simulink model "sampleModel1647"  (R2023a)
settings: Solver=VariableStepAuto  StartTime=0.0  StopTime=10.0  RelTol=1e-3
libraries: hdlsllib x7, simulink x4
settings Model: Creator=user1  LastModifiedBy=user1

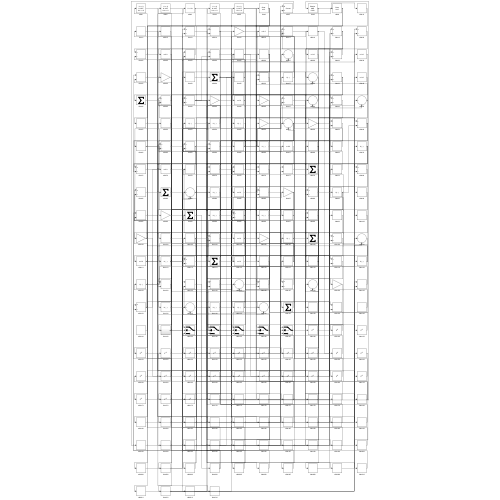
[thumbnail: Simulink's stored preview of the top-level diagram]
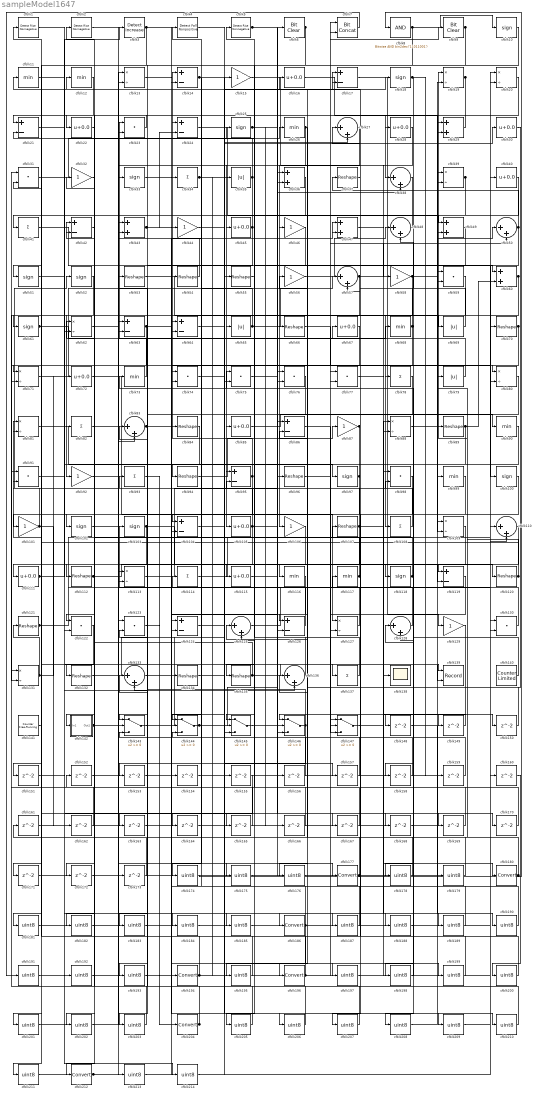
== system sampleModel1647 ==
  cfblk1 : hdlsllib/Logic and Bit Operations/Detect Rise Nonnegative  vinit=0  OutDataTypeStr=boolean
  cfblk{10,18,25,33,51..52,61,97,100,102..103,118} (12 alike) : Signum
  cfblk{15,32,44,46,56,58,87,92,101,106,129} (11 alike) : Gain
  cfblk{14,17,21,24,42,63..64,86,95,104,119,124,126} (13 alike) : Sum  Inputs=+-
  cfblk{16,22,28,30,40,45,67,72,85,105,111,115} (12 alike) : Bias  Bias=0.0  SaturateOnIntegerOverflow=off
  cfblk{37,53..55,66,70,84,89,94,96,107,112,120..121,132,134..135} (17 alike) : Reshape
  cfblk{34,41,78,82,93,108,114,137} (8 alike) : Sum  Inputs=+
  cfblk{13,19..20,39,62,71,80..81,88,109,113,127,131} (13 alike) : Product  Inputs=*/  RndMeth=Zero  SaturateOnIntegerOverflow=on
  cfblk{11..12,26,68,73,90,99,116..117} (9 alike) : MinMax
  cfblk{27,38,48,50,57,83,110,125,128,133,136} (11 alike) : Sum  Inputs=|++
  cfblk{23,31,59,74..77,91,98,122..123,130} (12 alike) : DotProduct  OutDataTypeStr=Inherit: Inherit via internal rule
  cfblk138 : Scope
  cfblk139 : Record  FileSettingsInternal="{\"entries\":[{\"content\":{\"excelSettings\":{\"content\":{},\"type\":\"Streamout.ExcelSettings\"}},\"type\":\"Streamout.FileSettingStorage\",\"uuid\":\"\"}],\"packageUris\":[\"http:\\/\\/schema.mathworks.com\\/mf0\\/streamout_blocks\\/R2020a\"],\"version\":\"1.0\"}"  Layout=[1 1]  SignalsInternal="{\"entries\":[{\"content\":{\"signals\":[{\"content\":{\"blockPath\":[],\"dimensions\":[1],\"domain\":\"\",\"lineColor\":\"#a2142f\",\"plots\":[1],\"port\":1,\"signalID\":2509,\"signalName\":\"XY Graph:1\"},\"type\":\"RecordBlkView.Signal\",\"uuid\":\"\"},{\"content\":{\"blockPath\":[],\"dimensions\":[1],\"domain\":\"\",\"lineColor\":\"#139fff\",\"plots\":[1],\"port\":2,\"signalID\":2512,\"signalName\":\"XY Graph:2\"},\"type\":\"RecordBlkView.Signal\",\"uuid\":\"\"}]},\"type\":\"RecordBlkView.InputSignals\",\"uuid\":\"\"}],\"packageUris\":[\"http:\\/\\/schema.mathworks.com\\/mf0\\/streamout_blocks\\/R2020a\"],\"version\":\"1.0\"}"  VisualizationBindings="{\"xyplotplugin\":{\"info\":[{\"series\":[{\"bindingParametersList\":[{\"parameter\":\"X-Axis\",\"signalID\":2509,\"signalName\":\"XY Graph:1\"},{\"parameter\":\"Y-Axis\",\"signalID\":2512,\"signalName\":\"XY Graph:2\"}],\"seriesID\":52686}],\"subplotID\":1}]}}"  CompatibilityTag=XY  st=-1
  cfblk140 : hdlsllib/Sources/Counter Limited  uplimit=7  tsamp=-1
  cfblk141 : hdlsllib/Sources/Counter Free-Running  NumBits=16  tsamp=-1
  cfblk142 : Subsystem
      settings: LibrarySourceBlock=|
      | hdlsllib/Ports &
      | Subsystems/Subsystem
  cfblk{143..147} (5 alike) : Switch  SaturateOnIntegerOverflow=off  InputSameDT=off
  cfblk{148..173} (26 alike) : Delay  SampleTime=1
  cfblk{174..176,178..179,181..185,187..193,195,197..203,205..211,213..214} (34 alike) : DataTypeConversion  OutDataTypeStr=uint8  SaturateOnIntegerOverflow=off  RndMeth=Floor
  cfblk{177,180,186,194,196,204,212} (7 alike) : DataTypeConversion  SaturateOnIntegerOverflow=off  RndMeth=Floor
  cfblk2 : hdlsllib/Logic and Bit Operations/Detect Rise Nonnegative  vinit=0  OutDataTypeStr=boolean
  cfblk{29,36,43,47,49,60} (6 alike) : Sum
  cfblk3 : simulink/Logic and Bit Operations/Detect Increase  vinit=0.0  OutDataTypeStr=boolean
      settings: LibrarySourceBlock=|
      | hdlsllib/Logic and Bit
      | Operations/Detect
      | Increase
  cfblk{35,65,69,79} (4 alike) : Abs  SaturateOnIntegerOverflow=off
  cfblk4 : hdlsllib/Logic and Bit Operations/Detect Fall Nonpositive  vinit=0  OutDataTypeStr=boolean
  cfblk5 : hdlsllib/Logic and Bit Operations/Detect Rise Nonnegative  vinit=0  OutDataTypeStr=boolean
  cfblk6 : simulink/Logic and Bit Operations/Bit Clear  iBit=0
      settings: LibrarySourceBlock=|
      | hdlsllib/Logic and Bit
      | Operations/Bit Clear
  cfblk7 : hdlsllib/Logic and Bit Operations/Bit Concat  numInputs=2
  cfblk8 : simulink/Logic and Bit Operations/Bitwise Operator  logicop=AND  UseBitMask=on  BitMask=bin2dec('11011001')  BitMaskRealWorld=Stored Integer
      settings: LibrarySourceBlock=|
      | hdlsllib/Logic and Bit
      | Operations/Bitwise
      | Operator
  cfblk9 : simulink/Logic and Bit Operations/Bit Clear  iBit=0
      settings: LibrarySourceBlock=|
      | hdlsllib/Logic and Bit
      | Operations/Bit Clear
  wires:
  cfblk17/1 -> cfblk129/1
  cfblk27/1 -> cfblk105/1
  cfblk61/1 -> cfblk68/1, cfblk165/1
  cfblk137/1 -> cfblk12/1
  cfblk60/1 -> cfblk108/1, cfblk178/1
  cfblk128/1 -> cfblk103/1
  cfblk35/1 -> cfblk21/2, cfblk164/1
  cfblk131/1 -> cfblk121/1, cfblk72/1
  cfblk30/1 -> cfblk125/1
  cfblk93/1 -> cfblk194/1
  cfblk88/1 -> cfblk19/1
  cfblk56/1 -> cfblk48/1
  cfblk26/1 -> cfblk106/1, cfblk126/1, cfblk43/2
  cfblk95/1 -> cfblk14/1, cfblk211/1
  cfblk48/1 -> cfblk45/1
  cfblk10/1 -> cfblk65/1
  cfblk135/1 -> cfblk139/1, cfblk42/2
  cfblk80/1 -> cfblk118/1
  cfblk28/1 -> cfblk88/2
  cfblk85/1 -> cfblk90/1
  cfblk101/1 -> cfblk52/1, cfblk162/1
  cfblk87/1 -> cfblk172/1, cfblk182/1
  cfblk19/1 -> cfblk38/1, cfblk128/2
  cfblk78/1 -> cfblk143/1
  cfblk72/1 -> cfblk127/1
  cfblk133/1 -> cfblk177/1
  cfblk97/1 -> cfblk94/1, cfblk146/3
  cfblk146/1 -> cfblk83/1, cfblk193/1
  cfblk29/1 -> cfblk28/1
  cfblk36/1 -> cfblk102/1
  cfblk141/1 -> cfblk81/1
  cfblk107/1 -> cfblk81/2, cfblk120/1, cfblk176/1
  cfblk106/1 -> cfblk143/2
  cfblk50/1 -> cfblk37/1, cfblk198/1
  cfblk125/1 -> cfblk117/1
  cfblk121/1 -> cfblk86/1, cfblk70/1
  cfblk18/1 -> cfblk158/1, cfblk159/1
  cfblk102/1 -> cfblk57/1
  cfblk94/1 -> cfblk87/1
  cfblk104/1 -> cfblk15/1
  cfblk54/1 -> cfblk23/1
  cfblk89/1 -> cfblk112/1, cfblk60/2, cfblk122/2
  cfblk68/1 -> cfblk92/1, cfblk11/1, cfblk71/2
  cfblk81/1 -> cfblk97/1
  cfblk124/1 -> cfblk27/2
  cfblk113/1 -> cfblk6/1
  cfblk103/1 -> cfblk116/1, cfblk122/1
  cfblk127/1 -> cfblk114/1
  cfblk24/1 -> cfblk58/1
  cfblk42/1 -> cfblk2/1
  cfblk143/1 -> cfblk18/1
  cfblk76/1 -> cfblk135/1
  cfblk118/1 -> cfblk16/1, cfblk208/1
  cfblk126/1 -> cfblk5/1
  cfblk73/1 -> cfblk23/2
  cfblk75/1 -> cfblk36/1
  cfblk39/1 -> cfblk113/2, cfblk148/1
  cfblk114/1 -> cfblk40/1
  cfblk15/1 -> cfblk138/1
  cfblk115/1 -> cfblk67/1
  cfblk37/1 -> cfblk17/1
  cfblk44/1 -> cfblk186/1
  cfblk112/1 -> cfblk119/1, cfblk83/2
  cfblk90/1 -> cfblk132/1
  cfblk46/1 -> cfblk115/1
  cfblk77/1 -> cfblk180/1
  cfblk123/1 -> cfblk204/1
  cfblk34/1 -> cfblk96/1, cfblk170/1, cfblk197/1
  cfblk20/1 -> cfblk212/1
  cfblk58/1 -> cfblk50/1, cfblk195/1
  cfblk105/1 -> cfblk63/1, cfblk111/1, cfblk47/2
  cfblk132/1 -> cfblk30/1
  cfblk119/1 -> cfblk127/2
  cfblk136/1 -> cfblk75/1
  cfblk71/1 -> cfblk34/1
  cfblk49/1 -> cfblk85/1
  cfblk16/1 -> cfblk109/1
  cfblk41/1 -> cfblk100/1
  cfblk96/1 -> cfblk119/2
  cfblk108/1 -> cfblk42/1
  cfblk130/1 -> cfblk17/2
  cfblk111/1 -> cfblk3/1, cfblk214/1
  cfblk14/1 -> cfblk144/1, cfblk66/1
  cfblk66/1 -> cfblk78/1
  cfblk12/1 -> cfblk22/1
  cfblk43/1 -> cfblk126/2, cfblk145/3, cfblk24/2, cfblk168/1
  cfblk23/1 -> cfblk21/1
  cfblk8/1 -> cfblk10/1, cfblk62/2
  cfblk22/1 -> cfblk142/1(In1)
  cfblk69/1 -> cfblk48/2
  cfblk45/1 -> cfblk41/1, cfblk163/1
  cfblk144/1 -> cfblk76/1, cfblk157/1
  cfblk100/1 -> cfblk101/1
  cfblk62/1 -> cfblk33/1
  cfblk91/1 -> cfblk136/2
  cfblk31/1 -> cfblk24/1
  cfblk4/1 -> cfblk137/1
  cfblk65/1 -> cfblk4/1, cfblk9/1, cfblk50/2
  cfblk57/1 -> cfblk104/1, cfblk131/2, cfblk49/2, cfblk145/2
  cfblk3/1 -> cfblk60/1, cfblk61/1
  cfblk79/1 -> cfblk53/1
  cfblk92/1 -> cfblk26/1
  cfblk67/1 -> cfblk104/2
  cfblk98/1 -> cfblk196/1
  cfblk116/1 -> cfblk124/2
  cfblk52/1 -> cfblk82/1
  cfblk83/1 -> cfblk47/1, cfblk210/1
  cfblk86/1 -> cfblk147/3
  cfblk140/1 -> cfblk73/1
  cfblk38/1 -> cfblk46/1
  cfblk109/1 -> cfblk144/2
  cfblk53/1 -> cfblk69/1
  cfblk40/1 -> cfblk95/1
  cfblk120/1 -> cfblk89/1, cfblk31/2
  cfblk5/1 -> cfblk38/2, cfblk49/1
  cfblk142/1(Out1) -> cfblk54/1, cfblk62/1, cfblk185/1
  cfblk6/1 -> cfblk51/1, cfblk201/1, cfblk203/1
  cfblk25/1 -> cfblk166/1, cfblk167/1
  cfblk63/1 -> cfblk80/2, cfblk151/1
  cfblk55/1 -> cfblk145/1
  cfblk51/1 -> cfblk139/2
  cfblk117/1 -> cfblk95/2, cfblk25/1
  cfblk70/1 -> cfblk109/2, cfblk71/1, cfblk80/1
  cfblk9/1 -> cfblk14/2, cfblk76/2
  cfblk129/1 -> cfblk149/1
  cfblk149/1 -> cfblk146/1
  cfblk47/1 -> cfblk150/1
  cfblk150/1 -> cfblk86/2
  cfblk152/1 -> cfblk147/1
  cfblk84/1 -> cfblk153/1
  cfblk33/1 -> cfblk154/1
  cfblk154/1 -> cfblk39/1
  cfblk134/1 -> cfblk155/1
  cfblk145/1 -> cfblk156/1
  cfblk156/1 -> cfblk113/1
  cfblk157/1 -> cfblk63/2
  cfblk158/1 -> cfblk136/1
  cfblk159/1 -> cfblk128/1
  cfblk161/1 -> cfblk29/2
  cfblk162/1 -> cfblk131/1
  cfblk163/1 -> cfblk75/2
  cfblk164/1 -> cfblk88/1
  cfblk165/1 -> cfblk124/1
  cfblk166/1 -> cfblk125/2
  cfblk167/1 -> cfblk1/1
  cfblk168/1 -> cfblk19/2
  cfblk11/1 -> cfblk169/1
  cfblk169/1 -> cfblk27/1
  cfblk170/1 -> cfblk57/2
  cfblk122/1 -> cfblk171/1
  cfblk171/1 -> cfblk147/2
  cfblk172/1 -> cfblk36/2
  cfblk173/1 -> cfblk91/2
  cfblk59/1 -> cfblk174/1
  cfblk174/1 -> cfblk8/1
  cfblk82/1 -> cfblk175/1
  cfblk175/1 -> cfblk59/1
  cfblk176/1 -> cfblk59/2
  cfblk177/1 -> cfblk143/3, cfblk56/1
  cfblk178/1 -> cfblk133/1
  cfblk179/1 -> cfblk133/2
  cfblk180/1 -> cfblk79/1, cfblk146/2
  cfblk155/1 -> cfblk181/1
  cfblk181/1 -> cfblk77/1
  cfblk182/1 -> cfblk77/2
  cfblk110/1 -> cfblk183/1
  cfblk183/1 -> cfblk84/1
  cfblk21/1 -> cfblk184/1
  cfblk184/1 -> cfblk110/1
  cfblk185/1 -> cfblk110/2
  cfblk186/1 -> cfblk144/3, cfblk205/1
  cfblk1/1 -> cfblk187/1
  cfblk187/1 -> cfblk44/1
  cfblk74/1 -> cfblk188/1
  cfblk188/1 -> cfblk39/2
  cfblk147/1 -> cfblk189/1
  cfblk189/1 -> cfblk74/1
  cfblk148/1 -> cfblk190/1
  cfblk190/1 -> cfblk74/2
  cfblk7/1 -> cfblk191/1
  cfblk191/1 -> cfblk29/1
  cfblk151/1 -> cfblk192/1
  cfblk192/1 -> cfblk7/1
  cfblk193/1 -> cfblk7/2
  cfblk194/1 -> cfblk179/1, cfblk152/1, cfblk35/1
  cfblk195/1 -> cfblk93/1
  cfblk196/1 -> cfblk161/1, cfblk160/1
  cfblk197/1 -> cfblk98/1
  cfblk198/1 -> cfblk98/2
  cfblk13/1 -> cfblk199/1
  cfblk199/1 -> cfblk107/1
  cfblk160/1 -> cfblk200/1
  cfblk200/1 -> cfblk13/1
  cfblk201/1 -> cfblk13/2
  cfblk32/1 -> cfblk202/1
  cfblk202/1 -> cfblk173/1
  cfblk203/1 -> cfblk32/1
  cfblk204/1 -> cfblk43/1, cfblk91/1
  cfblk205/1 -> cfblk123/1
  cfblk153/1 -> cfblk206/1
  cfblk206/1 -> cfblk123/2
  cfblk99/1 -> cfblk207/1
  cfblk207/1 -> cfblk31/1
  cfblk208/1 -> cfblk99/1
  cfblk64/1 -> cfblk209/1
  cfblk209/1 -> cfblk130/1
  cfblk210/1 -> cfblk64/1
  cfblk211/1 -> cfblk64/2
  cfblk212/1 -> cfblk130/2, cfblk55/1, cfblk134/1
  cfblk2/1 -> cfblk213/1
  cfblk213/1 -> cfblk20/1
  cfblk214/1 -> cfblk20/2

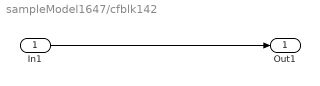
== system sampleModel1647/cfblk142 ==
  In1 : Inport
  Out1 : Outport
  wires:
  In1/1 -> Out1/1
